simulink model "radiator_simsc"  (R2016b)
settings: Solver=VariableStepAuto  StartTime=0.0  StopTime=10.0  RelTol=1e-3
libraries: fl_lib x10, nesl_utility x3
settings Model: Creator=gylaszlo  LastModifiedBy=gylaszlo

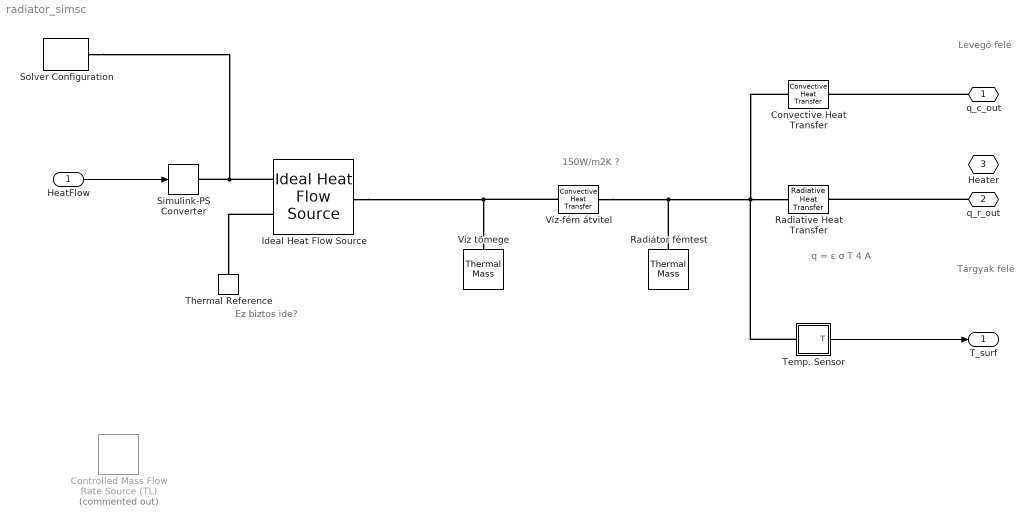
== system radiator_simsc ==
  note: q = ε σ T 4 A
  note: 150W/m2K ?
  note: Tárgyak felé
  note: Levegő felé
  note: Ez biztos ide?
  HeatFlow : Inport
  Controlled Mass Flow Rate Source (TL) : fl_lib/Thermal Liquid/Sources/Controlled Mass Flow Rate Source (TL)  Commented=on  area=0.01 m^2  length=0.1 m
  Convective Heat Transfer : fl_lib/Thermal/Thermal Elements/Convective Heat Transfer  area=area_radiator m^2  heat_tr_coeff=heat_transfer_convective_radiator W/(m^2 * K)  Q_specify=off  Q_priority=None  Q=0 J/s  T_specify=off  T_priority=None  T=0 K
  Ideal Heat Flow Source : fl_lib/Thermal/Thermal Sources/Ideal Heat Flow Source
  Radiative Heat Transfer : fl_lib/Thermal/Thermal Elements/Radiative Heat Transfer  area=area_radiator m^2  rad_tr_coeff=heat_transfer_radiant_radiator W/(m^2*K^4)  Q_specify=off  Q_priority=None  Q=0 J/s  T_specify=off  T_priority=None  T=0 K
  Radiátor fémtest : fl_lib/Thermal/Thermal Elements/Thermal Mass  mass=1 kg  sp_heat=447 J/kg/K  T_specify=off  T_priority=High  T=300 K  Q_specify=off  Q_priority=None  Q=0 J/s
  Simulink-PS Converter : nesl_utility/Simulink-PS Converter  PhysicalDomain=network_engine_domain  SubClassName=ps_input  LeftPortType=input  RightPortType=output  PseudoPeriodic=off  Frequencies=[]  NoiseDistribution=none  NoiseParameters=[]  Unit=1  AffineConversion=off  InputFiltering=off  SimscapeFilterOrder=1  InputFilterTimeConstant=0.001  UdotUserProvided=1
  Solver Configuration : nesl_utility/Solver Configuration  PhysicalDomain=network_engine_domain  SubClassName=solver  LeftPortType=input  RightPortType=generic  Accelerate=off  Tones=[]  Harmonics=[]  SimulateNoise=off  Profile=off  UseLocalSampling=off  EnableSwitchedLinearOptims=on  FrequencyDomain=off  UseCCode=off  RelTol=0.001  AbsTol=1e-06  MinStep=1e-09  ToWorkspace=off  RevertToSquareIcSolve=off  NumHomotopyIterations=100  PhasorMode=off  PhasorModeNumHarmonics=1  OverrideAbsTol=off  DoDC=off  ResidualTolerance=1e-09  UseLocalSolver=off  LocalSolverChoice=NE_BACKWARD_EULER_ADVANCER  LocalSolverSampleTime=0.001  DoFixedCost=off  MaxNonlinIter=3  MaxModeIter=2  LinearAlgebra=Sparse  DelaysMemoryBudget=1024  AutomaticFiltering=on  FilteringTimeConstant=0.001
  Temp. Sensor : Subsystem
  Thermal Reference : fl_lib/Thermal/Thermal Elements/Thermal Reference
  Víz tömege : fl_lib/Thermal/Thermal Elements/Thermal Mass  mass=1 kg  sp_heat=447 J/kg/K  T_specify=off  T_priority=High  T=300 K  Q_specify=off  Q_priority=None  Q=0 J/s
  Víz-fém átvitel : fl_lib/Thermal/Thermal Elements/Convective Heat Transfer  area=area_radiator m^2  heat_tr_coeff=heat_transfer_water_radiator W/(m^2 * K)  Q_specify=off  Q_priority=None  Q=0 J/s  T_specify=off  T_priority=None  T=0 K
  q_c_out : PMIOPort  Port=1  Side=Right
  q_r_out : PMIOPort  Port=2  Side=Right
  Heater : PMIOPort  Tag=PMCPort  Port=3  Side=Left
  T_surf : Outport
  wires:
  HeatFlow/1 -> Simulink-PS Converter/1
  Temp. Sensor/1(T) -> T_surf/1
  connections:
  Ideal Heat Flow Source/RConn1 -- Simulink-PS Converter/RConn1 -- Solver Configuration/RConn1
  Ideal Heat Flow Source/RConn2 -- Thermal Reference/LConn1
  Radiátor fémtest/LConn1 -- Víz-fém átvitel/RConn1 -- Radiative Heat Transfer/LConn1 -- Convective Heat Transfer/LConn1 -- Temp. Sensor/LConn1
  Víz-fém átvitel/LConn1 -- Víz tömege/LConn1 -- Ideal Heat Flow Source/LConn1
  q_c_out/RConn1 -- Convective Heat Transfer/RConn1
  q_r_out/RConn1 -- Radiative Heat Transfer/RConn1

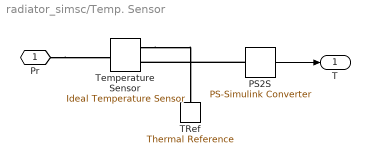
== system radiator_simsc/Temp. Sensor ==
  PS2S : nesl_utility/PS-Simulink Converter  PhysicalDomain=network_engine_domain  SubClassName=ps_output  LeftPortType=input  RightPortType=output  PseudoPeriodic=off  Frequencies=[]  Unit=degC  AffineConversion=on
  TRef : fl_lib/Thermal/Thermal Elements/Thermal Reference
  Temperature Sensor : fl_lib/Thermal/Thermal Sensors/Ideal Temperature Sensor
  Pr : PMIOPort  Port=1  Side=Left
  T : Outport
  wires:
  PS2S/1 -> T/1
  connections:
  Temperature Sensor/RConn1 -- TRef/LConn1
  PS2S/LConn1 -- Temperature Sensor/RConn2
  Pr/RConn1 -- Temperature Sensor/LConn1
